simulink model "linear_state_observer"  (R2022b)
settings: Solver=VariableStepAuto  StartTime=0.0  StopTime=10.0  RelTol=1e-3
settings Model: Creator=张倬境  LastModifiedBy=张倬境

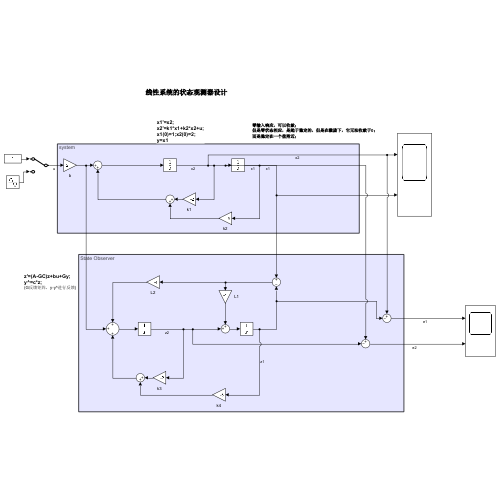
[thumbnail: Simulink's stored preview of the top-level diagram]
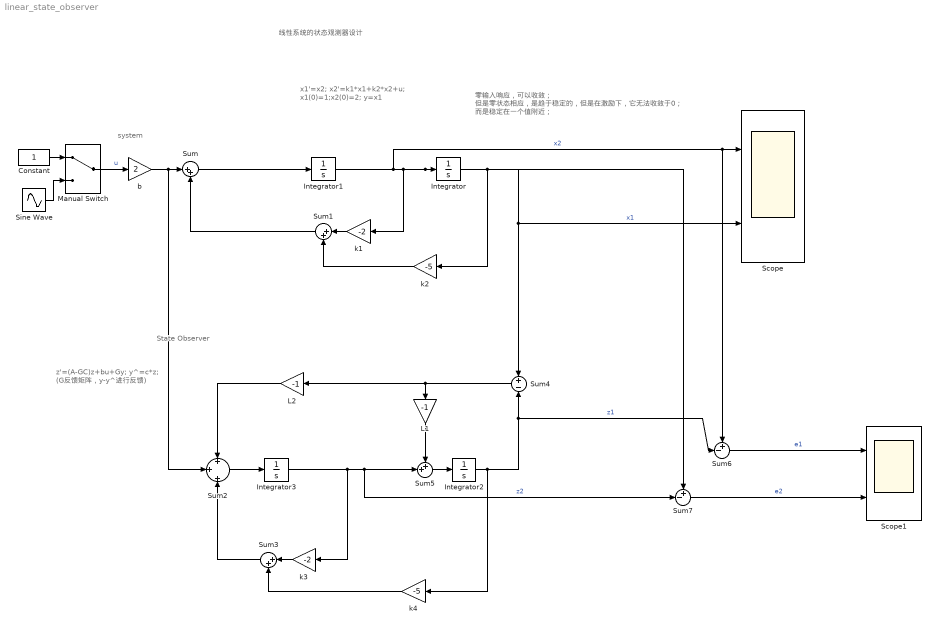
== system linear_state_observer ==
  note: system
  note: State Observer
  note: z'=(A-GC)z+bu+Gy;
      | y^=c*z;
      | (G反馈矩阵，y-y^进行反馈)
  note: 线性系统的状态观测器设计
  note: 零输入响应，可以收敛；
      | 但是零状态相应，是趋于稳定的，但是在激励下，它无法收敛于0；
      | 而是稳定在一个值附近；
  note: x1'=x2;
      | x2'=k1*x1+k2*x2+u;
      | x1(0)=1;x2(0)=2;
      | y=x1
  Constant : Constant
  Integrator : Integrator  InitialCondition=1
  Integrator1 : Integrator  InitialCondition=2
  Integrator2 : Integrator
  Integrator3 : Integrator
  L1 : Gain  Gain=-1
  L2 : Gain  Gain=-1
  Manual Switch : ManualSwitch
  Scope : Scope  NumInputPorts=2
  Scope1 : Scope  NumInputPorts=2
  Sine Wave : Sin  SampleTime=0
  Sum : Sum  Inputs=|++
  Sum1 : Sum  Inputs=|++
  Sum2 : Sum  Inputs=+|+|+
  Sum3 : Sum  Inputs=|++
  Sum4 : Sum  Inputs=+|-
  Sum5 : Sum  Inputs=++|
  Sum6 : Sum  Inputs=+-|
  Sum7 : Sum  Inputs=+-|
  b : Gain  Gain=2
  k1 : Gain  Gain=-2
  k2 : Gain  Gain=-5
  k3 : Gain  Gain=-2
  k4 : Gain  Gain=-5
  wires:
  Integrator1/1 -> Sum7/1, Integrator/1, k1/1, Sum6/1, Scope/1  "x2"
  Sum/1 -> Integrator1/1
  Integrator/1 -> Sum4/1, Scope/2, k2/1  "x1"
  k1/1 -> Sum1/1
  Sum1/1 -> Sum/2
  Constant/1 -> Manual Switch/1
  Sine Wave/1 -> Manual Switch/2
  k2/1 -> Sum1/2
  k4/1 -> Sum3/2
  Manual Switch/1 -> b/1  "u"
  Integrator2/1 -> k4/1, Sum4/2, Sum6/2  "z1"
  k3/1 -> Sum3/1
  Sum2/1 -> Integrator3/1
  Integrator3/1 -> k3/1, Sum7/2, Sum5/2  "z2"
  Sum4/1 -> L1/1, L2/1
  b/1 -> Sum2/2, Sum/1
  Sum3/1 -> Sum2/3
  L2/1 -> Sum2/1
  Sum5/1 -> Integrator2/1
  L1/1 -> Sum5/1
  Sum6/1 -> Scope1/1  "e1"
  Sum7/1 -> Scope1/2  "e2"
